simulink model "SchemSimulink"  (R2022a)
settings: Solver=VariableStepAuto  StartTime=0.0  StopTime=1.5  RelTol=1e-3
values from neighbouring files (symbols this model uses):
  C1 = minreal((1/Gzas) * (Gcl/ (1-Gcl)))    [Esercizio9_ContrAnalitico.m]    (also in Esercizio9_ContrDead.m; POSSIBILI_SPECIFICHE.m; myESE9_pt1.m; myESE9_pt2.m)
  C2 = minreal((1/Gzas) * (Gcl/ (1-Gcl)))    [myESE9_pt2.m]
  Gzas = tf(1, conv([1 -0.2],[1 -.01]), Tc)    [Esercizio9_ContrAnalitico.m]    (also in Esercizio9_ContrDead.m; POSSIBILI_SPECIFICHE.m; myESE9_pt1.m = tf(1, den, Tc); myESE9_pt2.m = Gzas*(z-3)*(-0.5))
  Tc = 0.01    [Esercizio9_ContrAnalitico.m]    (also in Esercizio9_ContrDead.m; POSSIBILI_SPECIFICHE.m; myESE9_pt1.m; myESE9_pt2.m)
settings Model: Creator=chiar  LastModifiedBy=Stefano
settings SolverCC: AlgebraicLoopSolver=TrustRegion
settings DebuggingCC: UnconnectedInputMsg=warning  UnconnectedOutputMsg=warning  UnconnectedLineMsg=warning  SFMachineParentedDataDiag=warning
settings RTWCC: DLArmComputeVersion=19.05

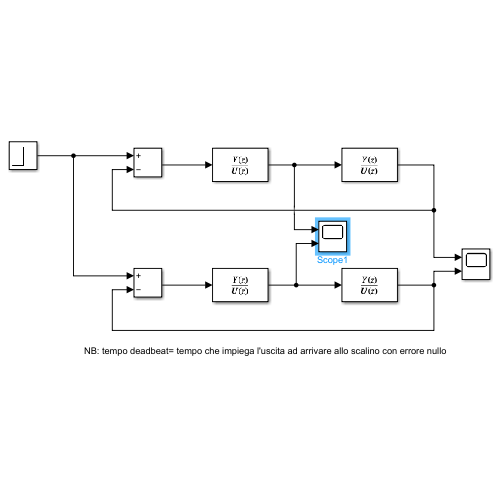
[thumbnail: Simulink's stored preview of the top-level diagram]
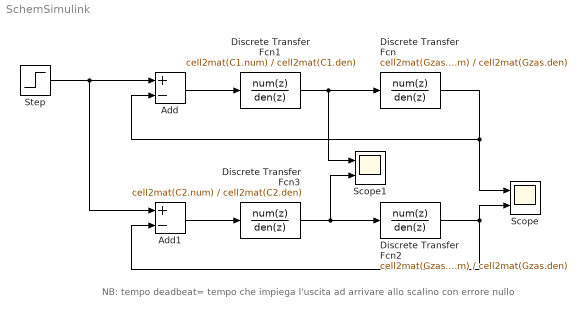
== system SchemSimulink ==
  note: NB: tempo deadbeat= tempo che impiega l'uscita ad arrivare allo scalino con errore nullo
  Add : Sum  Inputs=+-
  Add1 : Sum  Inputs=+-
  Discrete Transfer Fcn : DiscreteTransferFcn  Numerator=cell2mat(Gzas.num)  Denominator=cell2mat(Gzas.den)  SampleTime=Tc
  Discrete Transfer Fcn1 : DiscreteTransferFcn  Numerator=cell2mat(C1.num)  Denominator=cell2mat(C1.den)  SampleTime=Tc
  Discrete Transfer Fcn2 : DiscreteTransferFcn  Numerator=cell2mat(Gzas.num)  Denominator=cell2mat(Gzas.den)  SampleTime=Tc
  Discrete Transfer Fcn3 : DiscreteTransferFcn  Numerator=cell2mat(C2.num)  Denominator=cell2mat(C2.den)  SampleTime=Tc
  Scope : Scope  NumInputPorts=2
  Scope1 : Scope  NumInputPorts=2
  Step : Step  SampleTime=0
  wires:
  Step/1 -> Add1/1, Add/1
  Add/1 -> Discrete Transfer Fcn1/1
  Discrete Transfer Fcn1/1 -> Scope1/1, Discrete Transfer Fcn/1
  Discrete Transfer Fcn/1 -> Add/2, Scope/1
  Discrete Transfer Fcn2/1 -> Add1/2, Scope/2
  Add1/1 -> Discrete Transfer Fcn3/1
  Discrete Transfer Fcn3/1 -> Scope1/2, Discrete Transfer Fcn2/1
